simulink model "gear_logic_on_stm32"  (R2023a)
settings: Solver=FixedStepAuto  StartTime=0.0  StopTime=50  FixedStep=0.01  RelTol=1e-3  EnableMultiTasking=on
model workspace (MAT data in the model file):
  Var = 0
  downtab = [0  5  20  35; 0  5  20  35; 0  5  25  40; 0  5  30  50; 0  30  50  80; 0  30  50  80]
  downth = [0; 5; 40; 50; 90; 100]
  uptab = [10  30  50  1000000; 10  30  50  1000000; 15  30  50  1000000; 23  41  60  1000000; 40  70  100  1000000; 40  70  100  1000000]
  upth = [0; 25; 35; 50; 90; 100]
libraries: mbedblockslib x2
settings Model: SimulationMode=external  ExtModeTrigDuration=10  Creator=sgirardi  LastModifiedBy=atarsi
settings OptimizationCC: EnhancedBackFolding=on  PassReuseOutputArgsAs=Individual arguments  ZeroExternalMemoryAtStartup=off  ZeroInternalMemoryAtStartup=off  MaxStackSize=64  OptimizeBlockOrder=speed  DifferentSizesBufferReuse=on  OptimizationCustomize=off  EfficientTunableParamExpr=on
settings DebuggingCC: ParameterTunabilityLossMsg=error  UnconnectedInputMsg=warning  UnconnectedOutputMsg=warning  UnconnectedLineMsg=warning  UniqueDataStoreMsg=error
settings HardwareCC: ProdBitPerPointer=32  ProdBitPerSizeT=32  ProdBitPerPtrDiffT=32  ProdLargestAtomicInteger=Long  ProdLargestAtomicFloat=Double  ProdWordSize=32  ProdHWDeviceType=ARM Compatible->ARM Cortex
settings ModelReferenceCC: EnableRefExpFcnMdlSchedulingChecks=on
settings SFSimCC: MATLABDynamicMemAlloc=off
settings RTWCC: Description=Embedded Coder  SystemTargetFile=ert.tlc  HardwareBoard=STM32 Nucleo L476RG  TemplateMakefile=ert_default_tmf  Toolchain=GNU Tools for ARM Embedded Processors  DLArmComputeVersion=19.05
settings CodeAppCC: ForceParamTrailComments=on  IgnoreCustomStorageClasses=off  OperatorAnnotations=on  SimulinkDataObjDesc=on  SFDataObjDesc=on  InsertBlockDesc=on
settings ERTTargetCC: ExtMode=on  ExtModeTransport=3  ExtModeStaticAlloc=on  ExtModeStaticAllocSize=2000  ExtModeMexFile=ext_xcp  ExtModeMexArgs=1 3 115200  ExtModeIntrfLevel=Level2 - Open

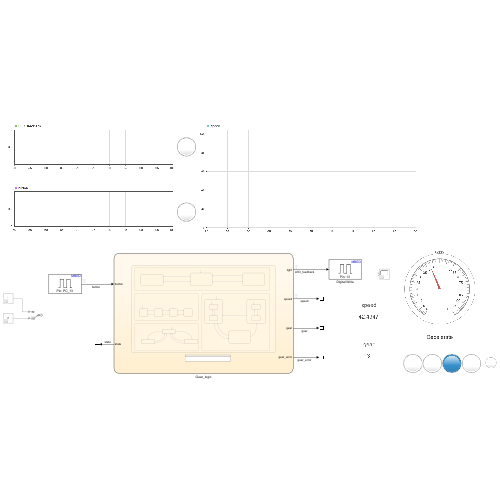
[thumbnail: Simulink's stored preview of the top-level diagram]
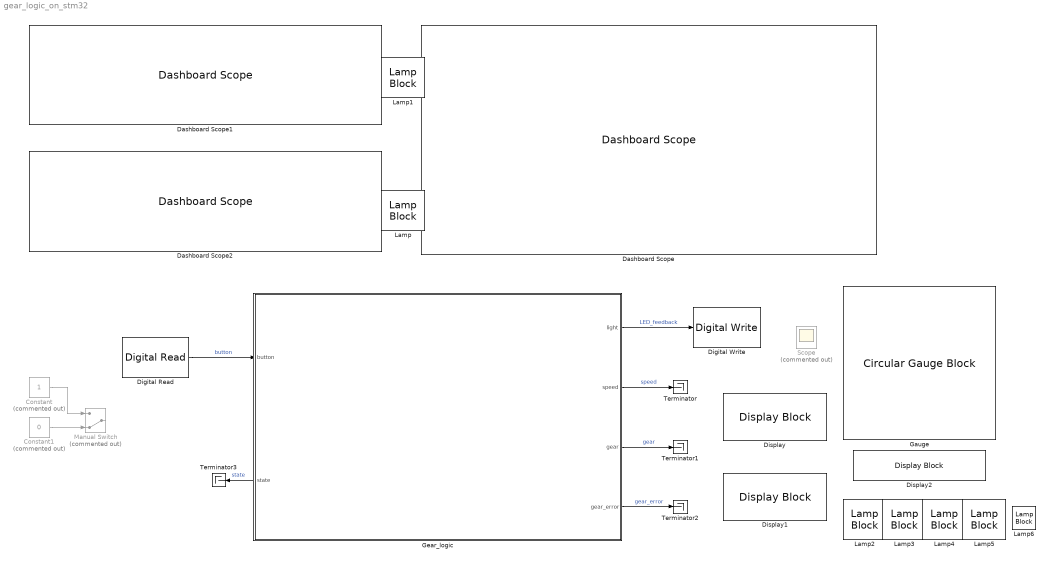
== system gear_logic_on_stm32 ==
  Constant : Constant  Commented=on
  Constant1 : Constant  Commented=on  Value=0
  Dashboard Scope : DashboardScope  Ymin=-0.5  Ymax=105  ScaleAtStop=off
  Dashboard Scope1 : DashboardScope  Ymin=-0.5  Ymax=1.5
  Dashboard Scope2 : DashboardScope  Ymin=-0.5  Ymax=1.5
  Digital Read : mbedblockslib/Digital Read  Pin=PC_13  Direction=input  SampleTime=-1
  Digital Write : mbedblockslib/Digital Write  Pin=13  Direction=output
  Display : DisplayBlock  Transparency=1  Opacity=0  ShowGrid=off
  Display1 : DisplayBlock  Transparency=1  Opacity=0  ShowGrid=off
  Display2 : DisplayBlock  LabelPosition=Hide  Format=long  Transparency=1
  Gauge : CircularGaugeBlock
  Gear_logic : Stateflow chart  TreatAsAtomicUnit=on
      settings: PortSchema="{\"entries\":[{\"content\":{\"sides\":[{\"content\":{\"connectorIds\":[\"In1\",\"Out5\"]},\"type\":\"ConnectorPlacement.EquallySpacedRectSide\",\"uuid\":\"fee7aec5-99ed-44e4-ae8a-3e054a8eb9e4\"},{\"content\":{\"connectorIds\":[\"Out1\",\"Out2\",\"Out3\",\"Out4\"],\"side\":\"RIGHT\"},\"type\":\"ConnectorPlacement.EquallySpacedRectSide\",\"uuid\":\"d017d7b8-a919-47a8-904c-65c4cd6a3d0b\"},{\"content\":{\"side\":\"TOP\"},\"type\":\"ConnectorPlacement.EquallySpacedRectSide\",\"uuid\":\"73b02b0d-2f13-4b10-9d89-8eae917eebf6\"}]},\"type\":\"ConnectorPlacement.EquallySpacedConnector\",\"uuid\":\"fd5e233b-a9b5-46bd-8666-79d703a5aac2\"}],\"packageUris\":[\"http://schema.mathworks.com/mf0/Connector/R2020b\"],\"version\":\"1.0\"}"
  Lamp{,1..6} (7 alike) : LampBlock  LabelPosition=Hide
  Manual Switch : ManualSwitch  Commented=on  CurrentSetting=0
  Scope : Scope  Commented=on
  Terminator{,1..3} (4 alike) : Terminator
  wires:
  Gear_logic/1(light) -> Digital Write/1  "LED_feedback"
  Digital Read/1 -> Gear_logic/1(button)  "button"
  Constant/1 -> Manual Switch/1
  Constant1/1 -> Manual Switch/2
  Gear_logic/2(speed) -> Terminator/1  "speed"
  Gear_logic/3(gear) -> Terminator1/1  "gear"
  Gear_logic/4(gear_error) -> Terminator2/1  "gear_error"
  Gear_logic/5(state) -> Terminator3/1  "state"

== stateflow chart gear_logic_on_stm32/Gear_logic ==
  settings: executeAtInitialization=1
  state gear_logic
    state move_state [parallel]
      settings: executionOrder=1
      state cruise
        entry:
        delta = 0;
        state="Cruise";
      state decel
        entry:
        delta = -0.08;
        state="Decelerate";
      state accel
        entry:
        delta = 0.08;
        state="Accelerate";
      (default) -> cruise
      decel -> cruise : [hasChangedTo(button, 0)]{scaleDown = 0;}
      cruise -> accel [order 2] : [hasChangedTo(button, 0) && scaleDown == 0]
      cruise -> decel [order 1] : [hasChangedTo(button, 0) && scaleDown ==  1]
      accel -> cruise : [hasChangedTo(button, 0)]{scaleDown = 1;}
    state gear_state [parallel]
      during:
      speed = max(0,min(speed+delta,100)-b*speed_tminus1);
      speed_tminus1=speed;
      settings: executionOrder=2
      state first
        entry:
        gear=1;
      state second
        entry:
        gear=2;
      state third
        entry:
        gear=3;
      state fourth
        entry:
        gear=4;
      (default) -> first
      first -> second : UP
      second -> third [order 1] : UP
      third -> fourth [order 1] : UP
      second -> first [order 2] : DOWN
      third -> second [order 2] : DOWN
      fourth -> third : DOWN
    state led_state [parallel]
      settings: executionOrder=3
      state blink_on_gear_change
        state OFF
          entry:
          light=0;
        state ON
          entry:
          light=1;
        (default) -> gear_logic.led_state.blink_on_gear_change.OFF
        gear_logic.led_state.blink_on_gear_change.ON -> gear_logic.led_state.blink_on_gear_change.OFF : after(0.05,sec)
        gear_logic.led_state.blink_on_gear_change.OFF -> gear_logic.led_state.blink_on_gear_change.ON : UP || DOWN
      state blinking
        state OFF
          entry:
          light=0;
          gear_error=0;
        state ON
          entry:
          light=1;
          gear_error=1;
        (default) -> gear_logic.led_state.blinking.OFF
        gear_logic.led_state.blinking.ON -> gear_logic.led_state.blinking.OFF : after(0.25,sec)
        gear_logic.led_state.blinking.OFF -> gear_logic.led_state.blinking.ON : after(0.25,sec)
      state prepare_to_blink
      (default) -> blink_on_gear_change
      blinking -> blink_on_gear_change : [delta <= 0]{gear_error=0;}
      blink_on_gear_change -> prepare_to_blink : [light == 0 && gear == 4 && speed >= up_th]
      prepare_to_blink -> blink_on_gear_change [order 2] : [gear < 4]
      prepare_to_blink -> blinking [order 1] : after(0.01,sec)
    state selection_state [parallel]
      during:
      computeThresholds();
      settings: executionOrder=4
      state steady_state
      state downshifting
      state upshifting
      (default) -> steady_state
      steady_state -> downshifting [order 2] : [speed < down_th]
      steady_state -> upshifting [order 1] : [speed > up_th]
      downshifting -> steady_state [order 2] : after(0.05, sec)
          | [speed <= down_th]
          | {send(DOWN, led_state);
          | send(DOWN, gear_state);}
      downshifting -> steady_state [order 1] : [speed > down_th]
      upshifting -> steady_state [order 2] : after(0.05, sec)
          | [speed >= up_th]
          | {send(UP,led_state);
          | send(UP,gear_state); }
      upshifting -> steady_state [order 1] : [speed < up_th]
  data: down_th local =0; up_th local =0; delta local =0; light output; scaleDown local =0; button input; speed output =0; gear output =1; gear_error output =0; b local =0.0003; speed_tminus1 local =0; state output string ="cruise"
  events: UP local FUNCTION_CALL_EVENT; DOWN local FUNCTION_CALL_EVENT
  function computeThresholds:
    | function computeThresholds
    |     
    |     % turn gear light on and set tachometer coefficients
    |     switch gear
    |         case 1
    |             down_th = 0;
    |             up_th = 10;
    |             rev = interp1([0 10],[0.5 6.5],speed,'pchip','extrap');
    |         case 2
    |             rev = interp1([5 10 30],[0.5 1 6.5],speed,'pchip','extrap');
    |             down_th = 10;
    |             up_th = 30;
    |         case 3
    |             rev = interp1([25 30 50],[0.5 1 6.5],speed,'pchip','extrap');
    |             down_th = 30;
    |             up_th = 70;
    |         case 4
    |             rev = interp1([40 50 100],[0.5 1 7],speed,'pchip','extrap');
    |             down_th = 70;
    |             up_th = 99;
    |     end
    | end
